simulink model "simwfs"  (Simulink 6.0)
settings: Solver=ode45  StartTime=0.0  StopTime=10.0  RelTol=1e-3
libraries: dspwin32 x3, dspsigops x1
settings Model: LastModifiedBy=fisbang

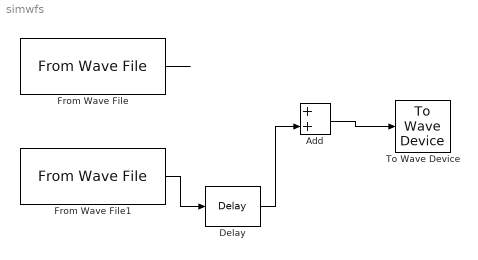
== system simwfs ==
  Add : Sum  OutScaling=2^-10
  Delay : dspsigops/Delay  dly_unit=Samples  delay=1  ic_detail=off  dif_ic_for_ch=off  dif_ic_for_dly=off  ic=0  reset_popup=None
  From Wave File : dspwin32/From Wave File  FileName=AA.wav  SamplesPerFrame=256  MinBufSize=256  dType=double  bLoop=off  timesToPlay=1  restartMode=immediately after last sample  firstSampleOutput=off  lastSampleOutput=off
  From Wave File1 : dspwin32/From Wave File  FileName=XX.wav  SamplesPerFrame=256  MinBufSize=256  dType=double  bLoop=off  timesToPlay=1  restartMode=immediately after last sample  firstSampleOutput=off  lastSampleOutput=off
  To Wave Device : dspwin32/To Wave Device  bufDuration=2  initDelay=0.1  useDefaultDevice=on  userDeviceID=Realtek AC97 Audio  enable24Bit=off
  wires:
  Add/1 -> To Wave Device/1
  From Wave File1/1 -> Delay/1
  Delay/1 -> Add/2
  From Wave File/1 -> ?
  ? -> Add/1
